simulink model "case9"  (R2024b)
settings: Solver=FixedStepAuto  StartTime=0  StopTime=1  FixedStep=1e-7  RelTol=1e-3
values from neighbouring files (symbols this model uses):
  SG_D_1_D = 0.01056    [IEEE9_case_parameters.m]    (also in case1_parameters.m; case2_parameters.m; case3_parameters.m; case4_parameters.m)
  SG_D_1_EnableSaturation = 0    [IEEE9_case_parameters.m]    (also in case1_parameters.m; case2_parameters.m; case3_parameters.m; case4_parameters.m)
  SG_D_1_f0 = 60    [IEEE9_case_parameters.m]    (also in case1_parameters.m; case2_parameters.m; case3_parameters.m; case4_parameters.m)
  SG_D_1_H = 7.5    [IEEE9_case_parameters.m]    (also in case1_parameters.m; case2_parameters.m; case3_parameters.m; case4_parameters.m)
  SG_D_1_K_A = 20    [IEEE9_case_parameters.m]    (also in case1_parameters.m; case2_parameters.m; case3_parameters.m; case4_parameters.m)
  SG_D_1_K_E = 1.000000e+1    (= 10)    [IEEE9_case_parameters.m]    (also in case1_parameters.m; case2_parameters.m; case3_parameters.m; case4_parameters.m)
  SG_D_1_K_F = 2.363    [IEEE9_case_parameters.m]    (also in case1_parameters.m; case2_parameters.m; case3_parameters.m; case4_parameters.m)
  SG_D_1_K_s = 0.5    [IEEE9_case_parameters.m]    (also in case1_parameters.m = 5; case2_parameters.m = 5; case3_parameters.m = 5; case4_parameters.m = 5)
  SG_D_1_R_a = 0.001088    [IEEE9_case_parameters.m]    (also in case1_parameters.m; case2_parameters.m; case3_parameters.m; case4_parameters.m)
  SG_D_1_S_A = 1    [IEEE9_case_parameters.m]    (also in case1_parameters.m; case2_parameters.m; case3_parameters.m; case4_parameters.m)
  SG_D_1_S_B = 0.103    [IEEE9_case_parameters.m]    (also in case1_parameters.m; case2_parameters.m; case3_parameters.m; case4_parameters.m)
  SG_D_1_S_N = 10.659857    [IEEE9_case_parameters.m]    (also in case1_parameters.m; case2_parameters.m; case3_parameters.m; case4_parameters.m)
  SG_D_1_SpeedPara = 200    [IEEE9_case_parameters.m]    (also in case1_parameters.m; case2_parameters.m; case3_parameters.m; case4_parameters.m)
  SG_D_1_T_0 = 0.720173    [IEEE9_case_parameters.m]    (also in case1_parameters.m = 0.755522; case2_parameters.m = 0.808931; case3_parameters.m = 0.869402; case4_parameters.m = 0.729316)
  SG_D_1_T_1 = 0.3    [IEEE9_case_parameters.m]    (also in case1_parameters.m; case2_parameters.m; case3_parameters.m; case4_parameters.m)
  SG_D_1_T_2 = 0.05    [IEEE9_case_parameters.m]    (also in case1_parameters.m; case2_parameters.m; case3_parameters.m; case4_parameters.m)
  SG_D_1_T_3 = 0.02    [IEEE9_case_parameters.m]    (also in case1_parameters.m; case2_parameters.m; case3_parameters.m; case4_parameters.m)
  SG_D_1_T_4 = 0.005    [IEEE9_case_parameters.m]    (also in case1_parameters.m; case2_parameters.m; case3_parameters.m; case4_parameters.m)
  SG_D_1_T_A = 0.02    [IEEE9_case_parameters.m]    (also in case1_parameters.m; case2_parameters.m; case3_parameters.m; case4_parameters.m)
  SG_D_1_T_dd = 8.000000e+0    (= 8)    [IEEE9_case_parameters.m]    (also in case1_parameters.m; case2_parameters.m; case3_parameters.m; case4_parameters.m)
  SG_D_1_T_ddd = 0.04    [IEEE9_case_parameters.m]    (also in case1_parameters.m; case2_parameters.m; case3_parameters.m; case4_parameters.m)
  SG_D_1_T_E = 0.314    [IEEE9_case_parameters.m]    (also in case1_parameters.m; case2_parameters.m; case3_parameters.m; case4_parameters.m)
  SG_D_1_T_F = 0.35    [IEEE9_case_parameters.m]    (also in case1_parameters.m; case2_parameters.m; case3_parameters.m; case4_parameters.m)
  SG_D_1_T_qd = 0.8    [IEEE9_case_parameters.m]    (also in case1_parameters.m; case2_parameters.m; case3_parameters.m; case4_parameters.m)
  SG_D_1_T_qdd = 0.02    [IEEE9_case_parameters.m]    (also in case1_parameters.m; case2_parameters.m; case3_parameters.m; case4_parameters.m)
  SG_D_1_T_speed = 0.1    [IEEE9_case_parameters.m]    (also in case1_parameters.m = 200; case2_parameters.m = 200; case3_parameters.m = 200; case4_parameters.m = 200)
  SG_D_1_T_w = 0.5    [IEEE9_case_parameters.m]    (also in case1_parameters.m; case2_parameters.m; case3_parameters.m; case4_parameters.m)
  SG_D_1_V_ref = 1.990276    [IEEE9_case_parameters.m]    (also in case1_parameters.m = 2.042296; case2_parameters.m = 2.051388; case3_parameters.m = 2.089584; case4_parameters.m = 2.01845)
  SG_D_1_w_ref = 376.991118    [IEEE9_case_parameters.m]    (also in case1_parameters.m; case2_parameters.m; case3_parameters.m; case4_parameters.m)
  SG_D_1_wb = 6.000000e+1    (= 60)    [IEEE9_case_parameters.m]    (also in case1_parameters.m; case2_parameters.m; case3_parameters.m; case4_parameters.m)
  SG_D_1_x_d = 1.9    [IEEE9_case_parameters.m]    (also in case1_parameters.m; case2_parameters.m; case3_parameters.m; case4_parameters.m)
  SG_D_1_x_dd = 0.302    [IEEE9_case_parameters.m]    (also in case1_parameters.m; case2_parameters.m; case3_parameters.m; case4_parameters.m)
  SG_D_1_x_ddd = 0.204    [IEEE9_case_parameters.m]    (also in case1_parameters.m; case2_parameters.m; case3_parameters.m; case4_parameters.m)
  SG_D_1_x_l = 0.05    [IEEE9_case_parameters.m]    (also in case1_parameters.m; case2_parameters.m; case3_parameters.m; case4_parameters.m)
  SG_D_1_x_q = 1.3    [IEEE9_case_parameters.m]    (also in case1_parameters.m; case2_parameters.m; case3_parameters.m; case4_parameters.m)
  SG_D_1_x_qd = 0.5    [IEEE9_case_parameters.m]    (also in case1_parameters.m; case2_parameters.m; case3_parameters.m; case4_parameters.m)
  SG_D_1_x_qdd = 0.3    [IEEE9_case_parameters.m]    (also in case1_parameters.m; case2_parameters.m; case3_parameters.m; case4_parameters.m)
  SG_D_2_D = 0.02    [IEEE9_case_parameters.m]    (also in case1_parameters.m; case2_parameters.m; case3_parameters.m; case4_parameters.m)
  SG_D_2_EnableSaturation = 0    [IEEE9_case_parameters.m]    (also in case1_parameters.m; case2_parameters.m; case3_parameters.m; case4_parameters.m)
  SG_D_2_f0 = 60    [IEEE9_case_parameters.m]    (also in case1_parameters.m; case2_parameters.m; case3_parameters.m; case4_parameters.m)
  SG_D_2_H = 8.000000e+0    (= 8)    [IEEE9_case_parameters.m]    (also in case1_parameters.m; case2_parameters.m; case3_parameters.m; case4_parameters.m)
  SG_D_2_K_A = 20    [IEEE9_case_parameters.m]    (also in case1_parameters.m; case2_parameters.m; case3_parameters.m; case4_parameters.m)
  SG_D_2_K_E = 1.000000e+1    (= 10)    [IEEE9_case_parameters.m]    (also in case1_parameters.m; case2_parameters.m; case3_parameters.m; case4_parameters.m)
  SG_D_2_K_F = 2.363    [IEEE9_case_parameters.m]    (also in case1_parameters.m; case2_parameters.m; case3_parameters.m; case4_parameters.m)
  SG_D_2_K_s = 0.5    [IEEE9_case_parameters.m]    (also in case1_parameters.m = 4; case2_parameters.m = 4; case3_parameters.m = 4; case4_parameters.m = 4)
  SG_D_2_R_a = 0.001088    [IEEE9_case_parameters.m]    (also in case1_parameters.m; case2_parameters.m; case3_parameters.m; case4_parameters.m)
  SG_D_2_S_A = 1    [IEEE9_case_parameters.m]    (also in case1_parameters.m; case2_parameters.m; case3_parameters.m; case4_parameters.m)
  SG_D_2_S_B = 0.103    [IEEE9_case_parameters.m]    (also in case1_parameters.m; case2_parameters.m; case3_parameters.m; case4_parameters.m)
  SG_D_2_S_N = 10.659857    [IEEE9_case_parameters.m]    (also in case1_parameters.m; case2_parameters.m; case3_parameters.m; case4_parameters.m)
  SG_D_2_SpeedPara = 200    [IEEE9_case_parameters.m]    (also in case1_parameters.m; case2_parameters.m; case3_parameters.m; case4_parameters.m)
  SG_D_2_T_0 = 1.632913    [IEEE9_case_parameters.m]    (also in case1_parameters.m = 1.632925; case2_parameters.m = 1.632915; case3_parameters.m = 1.632914; case4_parameters.m = 1.632927)
  SG_D_2_T_1 = 0.2    [IEEE9_case_parameters.m]    (also in case1_parameters.m; case2_parameters.m; case3_parameters.m; case4_parameters.m)
  SG_D_2_T_2 = 0.05    [IEEE9_case_parameters.m]    (also in case1_parameters.m; case2_parameters.m; case3_parameters.m; case4_parameters.m)
  SG_D_2_T_3 = 0.02    [IEEE9_case_parameters.m]    (also in case1_parameters.m; case2_parameters.m; case3_parameters.m; case4_parameters.m)
  SG_D_2_T_4 = 0.005    [IEEE9_case_parameters.m]    (also in case1_parameters.m; case2_parameters.m; case3_parameters.m; case4_parameters.m)
  SG_D_2_T_A = 0.02    [IEEE9_case_parameters.m]    (also in case1_parameters.m; case2_parameters.m; case3_parameters.m; case4_parameters.m)
  SG_D_2_T_dd = 7.9    [IEEE9_case_parameters.m]    (also in case1_parameters.m; case2_parameters.m; case3_parameters.m; case4_parameters.m)
  SG_D_2_T_ddd = 0.04    [IEEE9_case_parameters.m]    (also in case1_parameters.m; case2_parameters.m; case3_parameters.m; case4_parameters.m)
  SG_D_2_T_E = 0.314    [IEEE9_case_parameters.m]    (also in case1_parameters.m; case2_parameters.m; case3_parameters.m; case4_parameters.m)
  SG_D_2_T_F = 0.35    [IEEE9_case_parameters.m]    (also in case1_parameters.m; case2_parameters.m; case3_parameters.m; case4_parameters.m)
  SG_D_2_T_qd = 0.8    [IEEE9_case_parameters.m]    (also in case1_parameters.m; case2_parameters.m; case3_parameters.m; case4_parameters.m)
  SG_D_2_T_qdd = 0.015    [IEEE9_case_parameters.m]    (also in case1_parameters.m; case2_parameters.m; case3_parameters.m; case4_parameters.m)
  SG_D_2_T_speed = 0.1    [IEEE9_case_parameters.m]    (also in case1_parameters.m = 150; case2_parameters.m = 150; case3_parameters.m = 150; case4_parameters.m = 150)
  SG_D_2_T_w = 0.35    [IEEE9_case_parameters.m]    (also in case1_parameters.m; case2_parameters.m; case3_parameters.m; case4_parameters.m)
  SG_D_2_V_ref = 2.58547    [IEEE9_case_parameters.m]    (also in case1_parameters.m = 2.597896; case2_parameters.m = 2.587136; case3_parameters.m = 2.586042; case4_parameters.m = 2.599679)
  SG_D_2_w_ref = 376.991118    [IEEE9_case_parameters.m]    (also in case1_parameters.m; case2_parameters.m; case3_parameters.m; case4_parameters.m)
  SG_D_2_wb = 6.000000e+1    (= 60)    [IEEE9_case_parameters.m]    (also in case1_parameters.m; case2_parameters.m; case3_parameters.m; case4_parameters.m)
  SG_D_2_x_d = 1.8    [IEEE9_case_parameters.m]    (also in case1_parameters.m; case2_parameters.m; case3_parameters.m; case4_parameters.m)
  SG_D_2_x_dd = 0.302    [IEEE9_case_parameters.m]    (also in case1_parameters.m; case2_parameters.m; case3_parameters.m; case4_parameters.m)
  SG_D_2_x_ddd = 0.204    [IEEE9_case_parameters.m]    (also in case1_parameters.m; case2_parameters.m; case3_parameters.m; case4_parameters.m)
  SG_D_2_x_l = 0.05    [IEEE9_case_parameters.m]    (also in case1_parameters.m; case2_parameters.m; case3_parameters.m; case4_parameters.m)
  SG_D_2_x_q = 1.25    [IEEE9_case_parameters.m]    (also in case1_parameters.m; case2_parameters.m; case3_parameters.m; case4_parameters.m)
  SG_D_2_x_qd = 0.5    [IEEE9_case_parameters.m]    (also in case1_parameters.m; case2_parameters.m; case3_parameters.m; case4_parameters.m)
  SG_D_2_x_qdd = 0.3    [IEEE9_case_parameters.m]    (also in case1_parameters.m; case2_parameters.m; case3_parameters.m; case4_parameters.m)
  SG_D_3_D = 0.02    [IEEE9_case_parameters.m]    (also in case1_parameters.m; case2_parameters.m; case3_parameters.m; case4_parameters.m)
  SG_D_3_EnableSaturation = 0    [IEEE9_case_parameters.m]    (also in case1_parameters.m; case2_parameters.m; case3_parameters.m; case4_parameters.m)
  SG_D_3_f0 = 60    [IEEE9_case_parameters.m]    (also in case1_parameters.m; case2_parameters.m; case3_parameters.m; case4_parameters.m)
  SG_D_3_H = 7.7    [IEEE9_case_parameters.m]    (also in case1_parameters.m; case2_parameters.m; case3_parameters.m; case4_parameters.m)
  SG_D_3_K_A = 20    [IEEE9_case_parameters.m]    (also in case1_parameters.m; case2_parameters.m; case3_parameters.m; case4_parameters.m)
  SG_D_3_K_E = 1.000000e+1    (= 10)    [IEEE9_case_parameters.m]    (also in case1_parameters.m; case2_parameters.m; case3_parameters.m; case4_parameters.m)
  SG_D_3_K_F = 2.363    [IEEE9_case_parameters.m]    (also in case1_parameters.m; case2_parameters.m; case3_parameters.m; case4_parameters.m)
  SG_D_3_K_s = 0.2    [IEEE9_case_parameters.m]    (also in case1_parameters.m = 2; case2_parameters.m = 2; case3_parameters.m = 2; case4_parameters.m = 2)
  SG_D_3_R_a = 0.001088    [IEEE9_case_parameters.m]    (also in case1_parameters.m; case2_parameters.m; case3_parameters.m; case4_parameters.m)
  SG_D_3_S_A = 1    [IEEE9_case_parameters.m]    (also in case1_parameters.m; case2_parameters.m; case3_parameters.m; case4_parameters.m)
  SG_D_3_S_B = 0.103    [IEEE9_case_parameters.m]    (also in case1_parameters.m; case2_parameters.m; case3_parameters.m; case4_parameters.m)
  SG_D_3_S_N = 10.659857    [IEEE9_case_parameters.m]    (also in case1_parameters.m; case2_parameters.m; case3_parameters.m; case4_parameters.m)
  SG_D_3_SpeedPara = 200    [IEEE9_case_parameters.m]    (also in case1_parameters.m; case2_parameters.m; case3_parameters.m; case4_parameters.m)
  SG_D_3_T_0 = 0.850788    [IEEE9_case_parameters.m]    (also in case1_parameters.m = 0.850786; case2_parameters.m = 0.850787; case3_parameters.m; case4_parameters.m = 0.850786)
  SG_D_3_T_1 = 0.2    [IEEE9_case_parameters.m]    (also in case1_parameters.m; case2_parameters.m; case3_parameters.m; case4_parameters.m)
  SG_D_3_T_2 = 0.05    [IEEE9_case_parameters.m]    (also in case1_parameters.m; case2_parameters.m; case3_parameters.m; case4_parameters.m)
  SG_D_3_T_3 = 0.02    [IEEE9_case_parameters.m]    (also in case1_parameters.m; case2_parameters.m; case3_parameters.m; case4_parameters.m)
  SG_D_3_T_4 = 0.005    [IEEE9_case_parameters.m]    (also in case1_parameters.m; case2_parameters.m; case3_parameters.m; case4_parameters.m)
  SG_D_3_T_A = 0.02    [IEEE9_case_parameters.m]    (also in case1_parameters.m; case2_parameters.m; case3_parameters.m; case4_parameters.m)
  SG_D_3_T_dd = 8.1    [IEEE9_case_parameters.m]    (also in case1_parameters.m; case2_parameters.m; case3_parameters.m; case4_parameters.m)
  SG_D_3_T_ddd = 0.04    [IEEE9_case_parameters.m]    (also in case1_parameters.m; case2_parameters.m; case3_parameters.m; case4_parameters.m)
  SG_D_3_T_E = 0.314    [IEEE9_case_parameters.m]    (also in case1_parameters.m; case2_parameters.m; case3_parameters.m; case4_parameters.m)
  SG_D_3_T_F = 0.35    [IEEE9_case_parameters.m]    (also in case1_parameters.m; case2_parameters.m; case3_parameters.m; case4_parameters.m)
  SG_D_3_T_qd = 0.8    [IEEE9_case_parameters.m]    (also in case1_parameters.m; case2_parameters.m; case3_parameters.m; case4_parameters.m)
  SG_D_3_T_qdd = 0.015    [IEEE9_case_parameters.m]    (also in case1_parameters.m; case2_parameters.m; case3_parameters.m; case4_parameters.m)
  SG_D_3_T_speed = 0.1    [IEEE9_case_parameters.m]    (also in case1_parameters.m = 180; case2_parameters.m = 180; case3_parameters.m = 180; case4_parameters.m = 180)
  SG_D_3_T_w = 0.4    [IEEE9_case_parameters.m]    (also in case1_parameters.m; case2_parameters.m; case3_parameters.m; case4_parameters.m)
  SG_D_3_V_ref = 1.892727    [IEEE9_case_parameters.m]    (also in case1_parameters.m = 1.906439; case2_parameters.m = 1.895535; case3_parameters.m = 1.892105; case4_parameters.m = 1.906598)
  SG_D_3_w_ref = 376.991118    [IEEE9_case_parameters.m]    (also in case1_parameters.m; case2_parameters.m; case3_parameters.m; case4_parameters.m)
  SG_D_3_wb = 6.000000e+1    (= 60)    [IEEE9_case_parameters.m]    (also in case1_parameters.m; case2_parameters.m; case3_parameters.m; case4_parameters.m)
  SG_D_3_x_d = 1.85    [IEEE9_case_parameters.m]    (also in case1_parameters.m; case2_parameters.m; case3_parameters.m; case4_parameters.m)
  SG_D_3_x_dd = 0.302    [IEEE9_case_parameters.m]    (also in case1_parameters.m; case2_parameters.m; case3_parameters.m; case4_parameters.m)
  SG_D_3_x_ddd = 0.204    [IEEE9_case_parameters.m]    (also in case1_parameters.m; case2_parameters.m; case3_parameters.m; case4_parameters.m)
  SG_D_3_x_l = 0.05    [IEEE9_case_parameters.m]    (also in case1_parameters.m; case2_parameters.m; case3_parameters.m; case4_parameters.m)
  SG_D_3_x_q = 1.2    [IEEE9_case_parameters.m]    (also in case1_parameters.m; case2_parameters.m; case3_parameters.m; case4_parameters.m)
  SG_D_3_x_qd = 0.5    [IEEE9_case_parameters.m]    (also in case1_parameters.m; case2_parameters.m; case3_parameters.m; case4_parameters.m)
  SG_D_3_x_qdd = 0.3    [IEEE9_case_parameters.m]    (also in case1_parameters.m; case2_parameters.m; case3_parameters.m; case4_parameters.m)
(part 8 of 12)

== system case9/Apparatus/SG_D_2/d_psi_1d_SG_D_2_block ==
  note: d_psi_1d_SG_D_2 in case9
      | $-\frac{\psi _{\mathrm{1d},\mathrm{SG},D,2}-\psi _{\mathrm{fd},\mathrm{SG},D,2}+\frac{\left(x_{\mathrm{dd}}-x_{l}\right)\,\left(\frac{\psi _{\mathrm{1d},\mathrm{SG},D,2}\,\left(x_{\mathrm{dd}}-x_{\mathrm{ddd}}\right)}{x_{\mathrm{dd}}-x_{l}}-\psi _{d,\mathrm{SG},D,2}+\frac{\psi _{\mathrm{fd},\mathrm{SG},D,2}\,\left(x_{\mathrm{ddd}}-x_{l}\right)}{x_{\mathrm{dd}}-x_{l}}\right)}{x_{\mathrm{ddd}}}}{T_{\mathrm{ddd}}}$
      | Automatically generated on 2025-10-31 19:34:57 .
  State_psi_1d_SG_D_2_9b1ac : Inport
  State_psi_fd_SG_D_2_31ac8 : Inport  Port=2
  State_psi_1d_SG_D_2_4f306 : Inport  Port=3
  State_psi_d_SG_D_2_6c073 : Inport  Port=4
  State_psi_fd_SG_D_2_e2670 : Inport  Port=5
  Add_18fc3 : Sum
  Add_47703 : Sum
  Add_7959e : Sum
  Constant_-1_6db51 : Constant  Value=-1
  Constant_-1_c8e40 : Constant  Value=-1
  Constant_T_ddd_9bdcc : Constant  Value=T_ddd
  Constant_x_dd_6105a : Constant  Value=x_dd
  Constant_x_dd_8007f : Constant  Value=x_dd
  Constant_x_dd_b55d8 : Constant  Value=x_dd
  Constant_x_dd_ce09f : Constant  Value=x_dd
  Constant_x_ddd_0d417 : Constant  Value=x_ddd
  Constant_x_ddd_3c9c5 : Constant  Value=x_ddd
  Constant_x_ddd_7b55f : Constant  Value=x_ddd
  Constant_x_l_30dfb : Constant  Value=x_l
  Constant_x_l_5fcac : Constant  Value=x_l
  Constant_x_l_78aaf : Constant  Value=x_l
  Constant_x_l_b2922 : Constant  Value=x_l
  Divide_0f227 : Product  Inputs=*/
  Divide_c3476 : Product  Inputs=*/
  Divide_d66d9 : Product  Inputs=*/
  Divide_de240 : Product  Inputs=*/
  Product_030dc : Product
  Product_0f4d7 : Product
  Product_2a33a : Product
  Product_5af6c : Product
  Product_d701c : Product
  Subtract_1056e : Sum  Inputs=+-
  Subtract_1b7e0 : Sum  Inputs=+-
  Subtract_67225 : Sum  Inputs=+-
  Subtract_7c716 : Sum  Inputs=+-
  Subtract_a97c8 : Sum  Inputs=+-
  Subtract_cfbe6 : Sum  Inputs=+-
  Blockout_d_psi_1d_SG_D_2_4d013 : Outport
  wires:
  Subtract_67225/1 -> Product_5af6c/2
  Constant_x_l_b2922/1 -> Subtract_a97c8/2
  Divide_0f227/1 -> Add_47703/2
  Subtract_1b7e0/1 -> Product_d701c/2
  Constant_-1_c8e40/1 -> Product_0f4d7/1
  Constant_x_dd_8007f/1 -> Subtract_1056e/1
  Divide_c3476/1 -> Blockout_d_psi_1d_SG_D_2_4d013/1
  State_psi_fd_SG_D_2_31ac8/1 -> Add_7959e/2
  State_psi_1d_SG_D_2_4f306/1 -> Product_0f4d7/2
  Divide_de240/1 -> Subtract_1b7e0/2
  Constant_x_ddd_3c9c5/1 -> Subtract_1056e/2
  State_psi_1d_SG_D_2_9b1ac/1 -> Product_030dc/2
  Product_0f4d7/1 -> Product_2a33a/1
  Subtract_1056e/1 -> Product_2a33a/2
  Constant_x_dd_b55d8/1 -> Subtract_a97c8/1
  Constant_x_ddd_0d417/1 -> Subtract_67225/1
  Constant_x_l_5fcac/1 -> Subtract_67225/2
  Product_2a33a/1 -> Divide_d66d9/1
  Subtract_a97c8/1 -> Divide_d66d9/2
  State_psi_fd_SG_D_2_e2670/1 -> Product_5af6c/1
  Constant_x_dd_ce09f/1 -> Subtract_cfbe6/1
  Constant_x_l_78aaf/1 -> Subtract_7c716/2
  Constant_x_l_30dfb/1 -> Subtract_cfbe6/2
  Constant_x_ddd_7b55f/1 -> Divide_0f227/2
  Divide_d66d9/1 -> Add_18fc3/1
  State_psi_d_SG_D_2_6c073/1 -> Add_18fc3/2
  Product_5af6c/1 -> Divide_de240/1
  Subtract_cfbe6/1 -> Divide_de240/2
  Constant_x_dd_6105a/1 -> Subtract_7c716/1
  Add_18fc3/1 -> Subtract_1b7e0/1
  Constant_-1_6db51/1 -> Product_030dc/1
  Subtract_7c716/1 -> Product_d701c/1
  Product_030dc/1 -> Add_7959e/1
  Product_d701c/1 -> Divide_0f227/1
  Add_7959e/1 -> Add_47703/1
  Add_47703/1 -> Divide_c3476/1
  Constant_T_ddd_9bdcc/1 -> Divide_c3476/2

== system case9/Apparatus/SG_D_2/d_psi_d_SG_D_2_block ==
  note: d_psi_d_SG_D_2 in case9
      | $2\,\pi \,f_{0}\,\left(v_{d,\mathrm{SG},D,2}\,\sin\left(\theta _{\mathrm{SG},D,2}\right)-v_{q,\mathrm{SG},D,2}\,\cos\left(\theta _{\mathrm{SG},D,2}\right)+\frac{R_{a}\,\left(\frac{\psi _{\mathrm{1d},\mathrm{SG},D,2}\,\left(x_{\mathrm{dd}}-x_{\mathrm{ddd}}\right)}{x_{\mathrm{dd}}-x_{l}}-\psi _{d,\mathrm{SG},D,2}+\frac{\psi _{\mathrm{fd},\mathrm{SG},D,2}\,\left(x_{\mathrm{ddd}}-x_{l}\right)}{x_{\mathrm{dd}}-x_{l}}\right)}{x_{\mathrm{ddd}}}+\frac{\psi _{q,\mathrm{SG},D,2}\,w_{\mathrm{SG},D,2}}{2\,f_{0}\,\pi }\right)$
      | Automatically generated on 2025-10-31 19:34:54 .
  State_psi_1d_SG_D_2_d40cf : Inport
  State_psi_d_SG_D_2_25359 : Inport  Port=2
  State_psi_fd_SG_D_2_9b2f4 : Inport  Port=3
  Input_v_d_SG_D_2_d9ecd : Inport  Port=4
  State_theta_SG_D_2_7b7d1 : Inport  Port=5
  Input_v_q_SG_D_2_cb8d6 : Inport  Port=6
  State_theta_SG_D_2_ed5aa : Inport  Port=7
  State_psi_q_SG_D_2_78b00 : Inport  Port=8
  State_w_SG_D_2_fe89e : Inport  Port=9
  Add_1e130 : Sum
  Add_95736 : Sum
  Constant_-1_d1a72 : Constant  Value=-1
  Constant_-2.0_0a84b : Constant  Value=-2.0
  Constant_2.0_16524 : Constant  Value=2.0
  Constant_R_a_5fe79 : Constant  Value=R_a
  Constant_f0_c8b30 : Constant  Value=f0
  Constant_f0_d903e : Constant  Value=f0
  Constant_pi_38b7b : Constant  Value=pi
  Constant_pi_4bdac : Constant  Value=pi
  Constant_x_dd_2b82b : Constant  Value=x_dd
  Constant_x_dd_8fa44 : Constant  Value=x_dd
  Constant_x_dd_f8b5d : Constant  Value=x_dd
  Constant_x_ddd_0f6ba : Constant  Value=x_ddd
  Constant_x_ddd_d2d74 : Constant  Value=x_ddd
  Constant_x_ddd_e65f6 : Constant  Value=x_ddd
  Constant_x_l_65b5e : Constant  Value=x_l
  Constant_x_l_931b8 : Constant  Value=x_l
  Constant_x_l_af2d2 : Constant  Value=x_l
  Divide_2b745 : Product  Inputs=*/
  Divide_6bfed : Product  Inputs=*/
  Divide_c59a3 : Product  Inputs=*/
  Divide_ca9bb : Product  Inputs=*/
  MathFunc_cos_be2da : Trigonometry  Operator=cos
  MathFunc_sin_18cab : Trigonometry
  Product_0fb18 : Product
  Product_2a09d : Product
  Product_2f75e : Product
  Product_37f48 : Product
  Product_64ad8 : Product
  Product_6754d : Product
  Product_7a1cc : Product
  Product_a149a : Product
  Product_d38ff : Product
  Product_daf8b : Product
  Product_dd7d7 : Product
  Product_e1648 : Product
  Subtract_1b078 : Sum  Inputs=+-
  Subtract_24d92 : Sum  Inputs=+-
  Subtract_b40c2 : Sum  Inputs=+-
  Subtract_c682e : Sum  Inputs=+-
  Subtract_ccaed : Sum  Inputs=+-
  Subtract_e850a : Sum  Inputs=+-
  Subtract_f83ea : Sum  Inputs=+-
  Blockout_d_psi_d_SG_D_2_17d26 : Outport
  wires:
  MathFunc_sin_18cab/1 -> Product_e1648/2
  Constant_x_dd_f8b5d/1 -> Subtract_e850a/1
  Constant_-1_d1a72/1 -> Product_2f75e/1
  Constant_x_l_931b8/1 -> Subtract_e850a/2
  State_psi_1d_SG_D_2_d40cf/1 -> Product_2f75e/2
  Constant_f0_c8b30/1 -> Product_d38ff/2
  Constant_2.0_16524/1 -> Product_64ad8/1
  Constant_x_l_af2d2/1 -> Subtract_ccaed/2
  Constant_x_dd_2b82b/1 -> Subtract_24d92/1
  Product_2a09d/1 -> Blockout_d_psi_d_SG_D_2_17d26/1
  Constant_pi_38b7b/1 -> Product_64ad8/2
  Constant_x_ddd_e65f6/1 -> Subtract_24d92/2
  Subtract_1b078/1 -> Product_2a09d/2
  Product_2f75e/1 -> Product_6754d/1
  Product_64ad8/1 -> Product_7a1cc/1
  Subtract_24d92/1 -> Product_6754d/2
  Divide_ca9bb/1 -> Subtract_1b078/2
  Constant_x_ddd_d2d74/1 -> Subtract_b40c2/1
  Constant_x_l_65b5e/1 -> Subtract_b40c2/2
  Product_6754d/1 -> Divide_2b745/1
  Subtract_f83ea/1 -> Add_1e130/1
  Subtract_e850a/1 -> Divide_2b745/2
  State_psi_fd_SG_D_2_9b2f4/1 -> Product_daf8b/1
  Subtract_b40c2/1 -> Product_daf8b/2
  Constant_x_dd_8fa44/1 -> Subtract_ccaed/1
  Divide_2b745/1 -> Add_95736/1
  State_psi_d_SG_D_2_25359/1 -> Add_95736/2
  Product_daf8b/1 -> Divide_c59a3/1
  Subtract_ccaed/1 -> Divide_c59a3/2
  Add_95736/1 -> Subtract_c682e/1
  Divide_c59a3/1 -> Subtract_c682e/2
  Constant_R_a_5fe79/1 -> Product_0fb18/1
  Subtract_c682e/1 -> Product_0fb18/2
  Divide_6bfed/1 -> Subtract_f83ea/1
  State_theta_SG_D_2_7b7d1/1 -> MathFunc_sin_18cab/1
  Product_0fb18/1 -> Divide_6bfed/1
  Constant_-2.0_0a84b/1 -> Product_dd7d7/1
  Input_v_d_SG_D_2_d9ecd/1 -> Product_e1648/1
  Constant_x_ddd_0f6ba/1 -> Divide_6bfed/2
  State_theta_SG_D_2_ed5aa/1 -> MathFunc_cos_be2da/1
  Product_d38ff/1 -> Product_2a09d/1
  Product_e1648/1 -> Subtract_f83ea/2
  Product_dd7d7/1 -> Product_d38ff/1
  Input_v_q_SG_D_2_cb8d6/1 -> Product_37f48/1
  MathFunc_cos_be2da/1 -> Product_37f48/2
  State_psi_q_SG_D_2_78b00/1 -> Product_a149a/1
  State_w_SG_D_2_fe89e/1 -> Product_a149a/2
  Constant_f0_d903e/1 -> Product_7a1cc/2
  Constant_pi_4bdac/1 -> Product_dd7d7/2
  Product_37f48/1 -> Add_1e130/2
  Product_a149a/1 -> Divide_ca9bb/1
  Product_7a1cc/1 -> Divide_ca9bb/2
  Add_1e130/1 -> Subtract_1b078/1

== system case9/Apparatus/SG_D_2/d_psi_fd_SG_D_2_block ==
  note: d_psi_fd_SG_D_2 in case9
      | $-\frac{\psi _{\mathrm{fd},\mathrm{SG},D,2}-E_{\mathrm{fd},\mathrm{SG},D,2}+\left(x_{d}-x_{\mathrm{dd}}\right)\,\left(\frac{\frac{\psi _{\mathrm{1d},\mathrm{SG},D,2}\,\left(x_{\mathrm{dd}}-x_{\mathrm{ddd}}\right)}{x_{\mathrm{dd}}-x_{l}}-\psi _{d,\mathrm{SG},D,2}+\frac{\psi _{\mathrm{fd},\mathrm{SG},D,2}\,\left(x_{\mathrm{ddd}}-x_{l}\right)}{x_{\mathrm{dd}}-x_{l}}}{x_{\mathrm{ddd}}}-\frac{\left(x_{\mathrm{dd}}-x_{\mathrm{ddd}}\right)\,\left(\psi _{\mathrm{1d},\mathrm{SG},D,2}-\psi _{\mathrm{fd},\mathrm{SG},D,2}+\frac{\left(x_{\mathrm{dd}}-x_{l}\right)\,\left(\frac{\psi _{\mathrm{1d},\mathrm{SG},D,2}\,\left(x_{\mathrm{dd}}-x_{\mathrm{ddd}}\right)}{x_{\mathrm{dd}}-x_{l}}-\psi _{d,\mathrm{SG},D,2}+\frac{\psi _{\mathrm{fd},\mathrm{SG},D,2}\,\left(x_{\mathrm{ddd}}-x_{l}\right)}{x_{\mathrm{dd}}-x_{l}}\right)}{x_{\mathrm{ddd}}}\right)}{{\left(x_{\mathrm{dd}}-x_{l}\right)}^2}\right)}{T_{\mathrm{dd}}}$
      | Automatically generated on 2025-10-31 19:34:56 .
  State_E_fd_SG_D_2_5eccf : Inport
  State_psi_fd_SG_D_2_a7474 : Inport  Port=2
  State_psi_1d_SG_D_2_eaed7 : Inport  Port=3
  State_psi_fd_SG_D_2_5a6db : Inport  Port=4
  State_psi_1d_SG_D_2_c8d95 : Inport  Port=5
  State_psi_d_SG_D_2_a4024 : Inport  Port=6
  State_psi_fd_SG_D_2_151d3 : Inport  Port=7
  State_psi_1d_SG_D_2_fe5ae : Inport  Port=8
  State_psi_d_SG_D_2_cc219 : Inport  Port=9
  State_psi_fd_SG_D_2_1d8e3 : Inport  Port=10
  Add_676fd : Sum
  Add_809fa : Sum
  Constant_-1_955d1 : Constant  Value=-1
  Constant_-1_b7711 : Constant  Value=-1
  Constant_-1_bdc37 : Constant  Value=-1
  Constant_2.0_6795e : Constant  Value=2.0
  Constant_T_dd_c2ebe : Constant  Value=T_dd
  Constant_x_d_21a87 : Constant  Value=x_d
  Constant_x_dd_0c06f : Constant  Value=x_dd
  Constant_x_dd_1efb2 : Constant  Value=x_dd
  Constant_x_dd_3f41e : Constant  Value=x_dd
  Constant_x_dd_5792a : Constant  Value=x_dd
  Constant_x_dd_5f4b2 : Constant  Value=x_dd
  Constant_x_dd_657cb : Constant  Value=x_dd
  Constant_x_dd_687e3 : Constant  Value=x_dd
  Constant_x_dd_7842e : Constant  Value=x_dd
  Constant_x_dd_bf877 : Constant  Value=x_dd
  Constant_x_dd_d26d9 : Constant  Value=x_dd
  Constant_x_ddd_16458 : Constant  Value=x_ddd
  Constant_x_ddd_36004 : Constant  Value=x_ddd
  Constant_x_ddd_567b5 : Constant  Value=x_ddd
  Constant_x_ddd_7a9a3 : Constant  Value=x_ddd
  Constant_x_ddd_82ded : Constant  Value=x_ddd
  Constant_x_ddd_98200 : Constant  Value=x_ddd
  Constant_x_ddd_a2be3 : Constant  Value=x_ddd
  Constant_x_l_0f469 : Constant  Value=x_l
  Constant_x_l_13f2f : Constant  Value=x_l
  Constant_x_l_1c729 : Constant  Value=x_l
  Constant_x_l_2b70b : Constant  Value=x_l
  Constant_x_l_942a5 : Constant  Value=x_l
  Constant_x_l_ad6ed : Constant  Value=x_l
  Constant_x_l_b7b1d : Constant  Value=x_l
  Constant_x_l_c350b : Constant  Value=x_l
  Divide_290ff : Product  Inputs=*/
  Divide_583e5 : Product  Inputs=*/
  Divide_5f973 : Product  Inputs=*/
  Divide_6e344 : Product  Inputs=*/
  Divide_99481 : Product  Inputs=*/
  Divide_ce59d : Product  Inputs=*/
  Divide_d665e : Product  Inputs=*/
  Divide_fe53e : Product  Inputs=*/
  Power_5a083 : Math  Operator=pow
  Product_32dd5 : Product
  Product_34916 : Product
  Product_6c795 : Product
  Product_7516a : Product
  Product_7d71a : Product
  Product_a290e : Product
  Product_bd735 : Product
  Product_c09a7 : Product
  Product_e2bbc : Product
  Product_fd7d8 : Product
  Subtract_0377f : Sum  Inputs=+-
  Subtract_05f48 : Sum  Inputs=+-
  Subtract_1895f : Sum  Inputs=+-
  Subtract_1ab2a : Sum  Inputs=+-
  Subtract_1dd1f : Sum  Inputs=+-
  Subtract_3a82e : Sum  Inputs=+-
  Subtract_6ca6b : Sum  Inputs=+-
  Subtract_6db93 : Sum  Inputs=+-
  Subtract_74dc5 : Sum  Inputs=+-
  Subtract_8c2c0 : Sum  Inputs=+-
  Subtract_a2730 : Sum  Inputs=+-
  Subtract_a6d5d : Sum  Inputs=+-
  Subtract_aab37 : Sum  Inputs=+-
  Subtract_ad48d : Sum  Inputs=+-
  Subtract_bd0a5 : Sum  Inputs=+-
  Subtract_bf7ad : Sum  Inputs=+-
  Subtract_d44dc : Sum  Inputs=+-
  Subtract_df81d : Sum  Inputs=+-
  Subtract_fab20 : Sum  Inputs=+-
  Blockout_d_psi_fd_SG_D_2_bffd5 : Outport
  wires:
  Constant_x_dd_bf877/1 -> Subtract_1ab2a/1
  Constant_-1_b7711/1 -> Product_34916/1
  Constant_x_l_1c729/1 -> Subtract_8c2c0/2
  Divide_ce59d/1 -> Add_809fa/1
  Subtract_0377f/1 -> Product_7516a/2
  Constant_x_l_b7b1d/1 -> Subtract_1ab2a/2
  Product_7516a/1 -> Divide_6e344/1
  State_psi_1d_SG_D_2_c8d95/1 -> Product_34916/2
  Constant_x_dd_657cb/1 -> Subtract_6ca6b/1
  Product_c09a7/1 -> Divide_ce59d/1
  Constant_x_dd_0c06f/1 -> Subtract_ad48d/1
  Constant_x_ddd_7a9a3/1 -> Subtract_6ca6b/2
  Constant_x_dd_3f41e/1 -> Subtract_6db93/1
  Product_34916/1 -> Product_7d71a/1
  Subtract_6ca6b/1 -> Product_7d71a/2
  State_psi_d_SG_D_2_cc219/1 -> Add_809fa/2
  Constant_x_ddd_567b5/1 -> Subtract_0377f/1
  Constant_x_l_ad6ed/1 -> Subtract_0377f/2
  Product_7d71a/1 -> Divide_d665e/1
  Subtract_1ab2a/1 -> Divide_d665e/2
  State_psi_fd_SG_D_2_151d3/1 -> Product_7516a/1
  Subtract_bd0a5/1 -> Product_e2bbc/2
  Constant_x_dd_5792a/1 -> Subtract_05f48/1
  Constant_x_l_942a5/1 -> Subtract_05f48/2
  Product_a290e/1 -> Product_e2bbc/1
  Divide_d665e/1 -> Add_676fd/1
  State_psi_d_SG_D_2_a4024/1 -> Add_676fd/2
  Subtract_05f48/1 -> Divide_6e344/2
  Constant_x_dd_5f4b2/1 -> Subtract_8c2c0/1
  Constant_x_ddd_36004/1 -> Subtract_1dd1f/1
  Add_676fd/1 -> Subtract_74dc5/1
  Divide_6e344/1 -> Subtract_74dc5/2
  Constant_-1_bdc37/1 -> Product_32dd5/1
  Product_fd7d8/1 -> Divide_99481/1
  State_psi_1d_SG_D_2_fe5ae/1 -> Product_32dd5/2
  Subtract_ad48d/1 -> Product_a290e/2
  Constant_x_dd_1efb2/1 -> Subtract_aab37/1
  Divide_99481/1 -> Subtract_a6d5d/2
  Constant_-1_955d1/1 -> Product_a290e/1
  Constant_x_ddd_98200/1 -> Subtract_aab37/2
  Constant_x_ddd_16458/1 -> Divide_fe53e/2
  Subtract_8c2c0/1 -> Product_6c795/1
  Subtract_74dc5/1 -> Product_6c795/2
  State_psi_fd_SG_D_2_5a6db/1 -> Subtract_1895f/2
  Product_32dd5/1 -> Product_c09a7/1
  Subtract_aab37/1 -> Product_c09a7/2
  Constant_2.0_6795e/1 -> Power_5a083/2
  State_psi_1d_SG_D_2_eaed7/1 -> Subtract_1895f/1
  Constant_x_dd_d26d9/1 -> Subtract_d44dc/1
  Subtract_1dd1f/1 -> Product_fd7d8/2
  Constant_x_l_13f2f/1 -> Subtract_d44dc/2
  Constant_x_l_c350b/1 -> Subtract_1dd1f/2
  Constant_x_ddd_82ded/1 -> Subtract_ad48d/2
  Subtract_6db93/1 -> Divide_99481/2
  Product_6c795/1 -> Divide_fe53e/1
  Subtract_d44dc/1 -> Divide_ce59d/2
  State_psi_fd_SG_D_2_1d8e3/1 -> Product_fd7d8/1
  Constant_x_l_2b70b/1 -> Subtract_6db93/2
  Constant_x_dd_687e3/1 -> Subtract_bf7ad/1
  Subtract_1895f/1 -> Subtract_bd0a5/1
  Divide_fe53e/1 -> Subtract_bd0a5/2
  Constant_x_l_0f469/1 -> Subtract_bf7ad/2
  Subtract_bf7ad/1 -> Power_5a083/1
  Add_809fa/1 -> Subtract_a6d5d/1
  Product_e2bbc/1 -> Divide_290ff/1
  Power_5a083/1 -> Divide_290ff/2
  Subtract_a6d5d/1 -> Divide_5f973/1
  Constant_x_ddd_a2be3/1 -> Divide_5f973/2
  Constant_x_d_21a87/1 -> Subtract_fab20/1
  Constant_x_dd_7842e/1 -> Subtract_fab20/2
  Divide_290ff/1 -> Subtract_3a82e/1
  Divide_5f973/1 -> Subtract_3a82e/2
  State_E_fd_SG_D_2_5eccf/1 -> Subtract_a2730/1
  State_psi_fd_SG_D_2_a7474/1 -> Subtract_a2730/2
  Subtract_fab20/1 -> Product_bd735/1
  Subtract_3a82e/1 -> Product_bd735/2
  Subtract_a2730/1 -> Subtract_df81d/1
  Product_bd735/1 -> Subtract_df81d/2
  Subtract_df81d/1 -> Divide_583e5/1
  Constant_T_dd_c2ebe/1 -> Divide_583e5/2
  Divide_583e5/1 -> Blockout_d_psi_fd_SG_D_2_bffd5/1

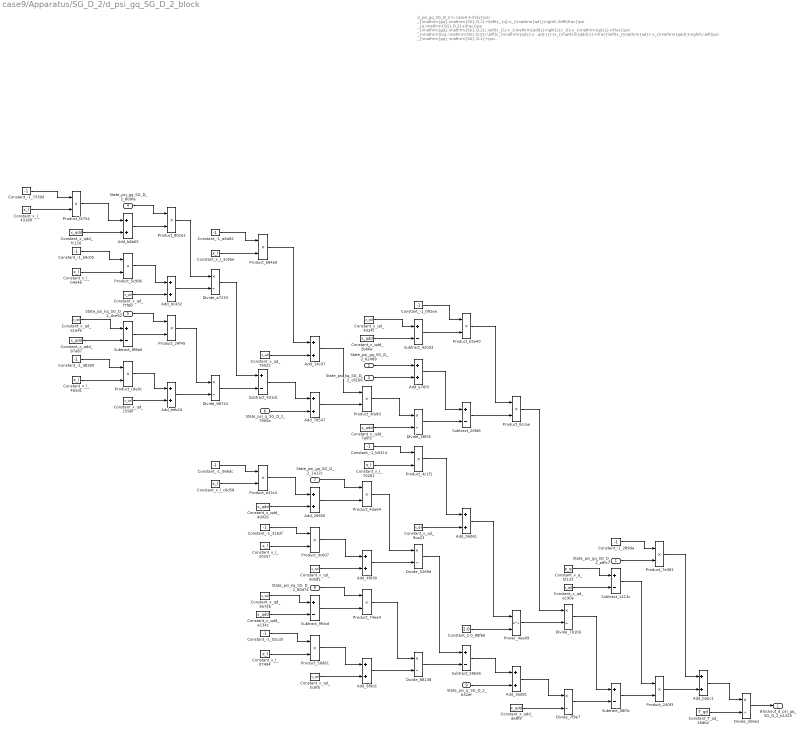
== system case9/Apparatus/SG_D_2/d_psi_gq_SG_D_2_block ==
  note: d_psi_gq_SG_D_2 in case9
      | $-\frac{\psi _{\mathrm{gq},\mathrm{SG},D,2}+\left(x_{q}-x_{\mathrm{qd}}\right)\,\left(\frac{\psi _{q,\mathrm{SG},D,2}+\frac{\psi _{\mathrm{gq},\mathrm{SG},D,2}\,\left(x_{l}-x_{\mathrm{qdd}}\right)}{x_{l}-x_{\mathrm{qd}}}+\frac{\psi _{\mathrm{kq},\mathrm{SG},D,2}\,\left(x_{\mathrm{qd}}-x_{\mathrm{qdd}}\right)}{x_{l}-x_{\mathrm{qd}}}}{x_{\mathrm{qdd}}}+\frac{\left(x_{\mathrm{qd}}-x_{\mathrm{qdd}}\right)\,\left(\psi _{\mathrm{gq},\mathrm{SG},D,2}+\psi _{\mathrm{kq},\mathrm{SG},D,2}+\frac{\left(x_{l}-x_{\mathrm{qd}}\right)\,\left(\psi _{q,\mathrm{SG},D,2}+\frac{\psi _{\mathrm{gq},\mathrm{SG},D,2}\,\left(x_{l}-x_{\mathrm{qdd}}\right)}{x_{l}-x_{\mathrm{qd}}}+\frac{\psi _{\mathrm{kq},\mathrm{SG},D,2}\,\left(x_{\mathrm{qd}}-x_{\mathrm{qdd}}\right)}{x_{l}-x_{\mathrm{qd}}}\right)}{x_{\mathrm{qdd}}}\right)}{{\left(x_{l}-x_{\mathrm{qd}}\right)}^2}\right)}{T_{\mathrm{qd}}}$
      | Automatically generated on 2025-10-31 19:34:58 .
  State_psi_gq_SG_D_2_a8fc7 : Inport
  State_psi_gq_SG_D_2_62489 : Inport  Port=2
  State_psi_kq_SG_D_2_c8166 : Inport  Port=3
  State_psi_gq_SG_D_2_800fa : Inport  Port=4
  State_psi_kq_SG_D_2_dce92 : Inport  Port=5
  State_psi_q_SG_D_2_7905a : Inport  Port=6
  State_psi_gq_SG_D_2_1a12c : Inport  Port=7
  State_psi_kq_SG_D_2_80d74 : Inport  Port=8
  State_psi_q_SG_D_2_b32ef : Inport  Port=9
  Add_06061 : Sum
  Add_14c97 : Sum
  Add_20850 : Sum
  Add_3ad81 : Sum
  Add_4f930 : Sum
  Add_6f9c6 : Sum
  Add_78547 : Sum
  Add_b8a05 : Sum
  Add_babc1 : Sum
  Add_dc432 : Sum
  Add_e76f3 : Sum
  Add_eeb16 : Sum
  Constant_-1_02cd3 : Constant  Value=-1
  Constant_-1_066dc : Constant  Value=-1
  Constant_-1_092ee : Constant  Value=-1
  Constant_-1_289da : Constant  Value=-1
  Constant_-1_3162f : Constant  Value=-1
  Constant_-1_7339d : Constant  Value=-1
  Constant_-1_a6a82 : Constant  Value=-1
  Constant_-1_b0314 : Constant  Value=-1
  Constant_-1_b9c05 : Constant  Value=-1
  Constant_-1_d8300 : Constant  Value=-1
  Constant_2.0_88f60 : Constant  Value=2.0
  Constant_T_qd_26db2 : Constant  Value=T_qd
  Constant_x_l_07494 : Constant  Value=x_l
  Constant_x_l_20257 : Constant  Value=x_l
  Constant_x_l_3c8be : Constant  Value=x_l
  Constant_x_l_43180 : Constant  Value=x_l
  Constant_x_l_4b5d1 : Constant  Value=x_l
  Constant_x_l_70261 : Constant  Value=x_l
  Constant_x_l_b454e : Constant  Value=x_l
  Constant_x_l_c0d58 : Constant  Value=x_l
  Constant_x_q_5f131 : Constant  Value=x_q
  Constant_x_qd_159ef : Constant  Value=x_qd
  Constant_x_qd_4324f : Constant  Value=x_qd
  Constant_x_qd_50591 : Constant  Value=x_qd
  Constant_x_qd_5c6fb : Constant  Value=x_qd
  Constant_x_qd_79022 : Constant  Value=x_qd
  Constant_x_qd_9a7eb : Constant  Value=x_qd
  Constant_x_qd_9ca23 : Constant  Value=x_qd
  Constant_x_qd_e190e : Constant  Value=x_qd
  Constant_x_qd_e1a4e : Constant  Value=x_qd
  Constant_x_qd_f7f60 : Constant  Value=x_qd
  Constant_x_qdd_2b66e : Constant  Value=x_qdd
  Constant_x_qdd_7a6f2 : Constant  Value=x_qdd
  Constant_x_qdd_97a87 : Constant  Value=x_qdd
  Constant_x_qdd_a134c : Constant  Value=x_qdd
  Constant_x_qdd_dd426 : Constant  Value=x_qdd
  Constant_x_qdd_de8f9 : Constant  Value=x_qdd
  Constant_x_qdd_fc116 : Constant  Value=x_qdd
  Divide_38f35 : Product  Inputs=*/
  Divide_5269d : Product  Inputs=*/
  Divide_7b1b6 : Product  Inputs=*/
  Divide_7f9e7 : Product  Inputs=*/
  Divide_88138 : Product  Inputs=*/
  Divide_98724 : Product  Inputs=*/
  Divide_a7233 : Product  Inputs=*/
  Divide_d56e2 : Product  Inputs=*/
  Power_4ea09 : Math  Operator=pow
  Product_0ccae : Product
  Product_240f3 : Product
  Product_24f45 : Product
  Product_3fa9d : Product
  Product_4c1f1 : Product
  Product_4da64 : Product
  Product_56d61 : Product
  Product_5c996 : Product
  Product_74ea4 : Product
  Product_7e381 : Product
  Product_802e2 : Product
  Product_a33c4 : Product
  Product_b5e40 : Product
  Product_b84a0 : Product
  Product_cde0c : Product
  Product_dc607 : Product
  Product_f4754 : Product
  Subtract_08f3c : Sum  Inputs=+-
  Subtract_1413c : Sum  Inputs=+-
  Subtract_20fd6 : Sum  Inputs=+-
  Subtract_420d3 : Sum  Inputs=+-
  Subtract_4d1dc : Sum  Inputs=+-
  Subtract_59b65 : Sum  Inputs=+-
  Subtract_8f8a0 : Sum  Inputs=+-
  Subtract_9fcbd : Sum  Inputs=+-
  Blockout_d_psi_gq_SG_D_2_b1325 : Outport
  wires:
  Constant_x_l_07494/1 -> Product_56d61/2
  Constant_x_l_c0d58/1 -> Product_a33c4/2
  Constant_x_qd_e1a4e/1 -> Subtract_8f8a0/1
  Constant_x_l_70261/1 -> Product_4c1f1/2
  Constant_x_qdd_2b66e/1 -> Subtract_420d3/2
  Constant_-1_d8300/1 -> Product_cde0c/1
  Constant_-1_7339d/1 -> Product_f4754/1
  State_psi_gq_SG_D_2_62489/1 -> Add_e76f3/1
  Constant_x_qdd_97a87/1 -> Subtract_8f8a0/2
  Constant_x_qd_4324f/1 -> Subtract_420d3/1
  Constant_x_l_4b5d1/1 -> Product_cde0c/2
  Constant_x_l_43180/1 -> Product_f4754/2
  Product_cde0c/1 -> Add_eeb16/1
  Product_f4754/1 -> Add_b8a05/1
  Constant_x_l_b454e/1 -> Product_5c996/2
  Constant_x_l_3c8be/1 -> Product_b84a0/2
  Constant_x_qd_159ef/1 -> Add_eeb16/2
  Constant_x_qdd_fc116/1 -> Add_b8a05/2
  Constant_-1_b9c05/1 -> Product_5c996/1
  Constant_x_qd_5c6fb/1 -> Add_6f9c6/2
  Constant_x_qdd_dd426/1 -> Add_20850/2
  State_psi_gq_SG_D_2_800fa/1 -> Product_802e2/1
  Add_eeb16/1 -> Divide_98724/2
  Add_b8a05/1 -> Product_802e2/2
  Constant_x_qd_e190e/1 -> Subtract_1413c/2
  Product_5c996/1 -> Add_dc432/1
  Constant_x_qd_f7f60/1 -> Add_dc432/2
  State_psi_kq_SG_D_2_dce92/1 -> Product_24f45/1
  Divide_a7233/1 -> Subtract_4d1dc/1
  Subtract_8f8a0/1 -> Product_24f45/2
  Product_802e2/1 -> Divide_a7233/1
  Add_dc432/1 -> Divide_a7233/2
  Add_78547/1 -> Product_3fa9d/2
  Product_24f45/1 -> Divide_98724/1
  Constant_-1_a6a82/1 -> Product_b84a0/1
  Divide_98724/1 -> Subtract_4d1dc/2
  Constant_-1_02cd3/1 -> Product_56d61/1
  Constant_-1_066dc/1 -> Product_a33c4/1
  Product_b84a0/1 -> Add_14c97/1
  Constant_x_qdd_a134c/1 -> Subtract_9fcbd/2
  Constant_x_qd_79022/1 -> Add_14c97/2
  Subtract_4d1dc/1 -> Add_78547/1
  Constant_-1_b0314/1 -> Product_4c1f1/1
  State_psi_q_SG_D_2_7905a/1 -> Add_78547/2
  Product_56d61/1 -> Add_6f9c6/1
  Product_a33c4/1 -> Add_20850/1
  Constant_-1_3162f/1 -> Product_dc607/1
  Product_3fa9d/1 -> Divide_38f35/1
  Constant_x_l_20257/1 -> Product_dc607/2
  Product_240f3/1 -> Add_babc1/2
  Constant_x_qd_9a7eb/1 -> Subtract_9fcbd/1
  Add_14c97/1 -> Product_3fa9d/1
  State_psi_gq_SG_D_2_1a12c/1 -> Product_4da64/1
  Add_6f9c6/1 -> Divide_88138/2
  Add_20850/1 -> Product_4da64/2
  Product_dc607/1 -> Add_4f930/1
  Constant_x_qd_50591/1 -> Add_4f930/2
  State_psi_kq_SG_D_2_80d74/1 -> Product_74ea4/1
  Subtract_9fcbd/1 -> Product_74ea4/2
  Divide_88138/1 -> Subtract_59b65/2
  State_psi_kq_SG_D_2_c8166/1 -> Add_e76f3/2
  Product_74ea4/1 -> Divide_88138/1
  Constant_x_qdd_7a6f2/1 -> Divide_38f35/2
  Product_4da64/1 -> Divide_5269d/1
  Add_4f930/1 -> Divide_5269d/2
  Constant_-1_092ee/1 -> Product_b5e40/1
  Subtract_420d3/1 -> Product_b5e40/2
  Add_e76f3/1 -> Subtract_20fd6/1
  Divide_38f35/1 -> Subtract_20fd6/2
  Product_4c1f1/1 -> Add_06061/1
  Constant_x_qd_9ca23/1 -> Add_06061/2
  Divide_5269d/1 -> Subtract_59b65/1
  Product_b5e40/1 -> Product_0ccae/1
  Subtract_20fd6/1 -> Product_0ccae/2
  Add_06061/1 -> Power_4ea09/1
  Constant_2.0_88f60/1 -> Power_4ea09/2
  Subtract_59b65/1 -> Add_3ad81/1
  State_psi_q_SG_D_2_b32ef/1 -> Add_3ad81/2
  Product_0ccae/1 -> Divide_7b1b6/1
  Power_4ea09/1 -> Divide_7b1b6/2
  Add_3ad81/1 -> Divide_7f9e7/1
  Constant_x_qdd_de8f9/1 -> Divide_7f9e7/2
  Constant_x_q_5f131/1 -> Subtract_1413c/1
  Divide_7b1b6/1 -> Subtract_08f3c/1
  Divide_7f9e7/1 -> Subtract_08f3c/2
  Divide_d56e2/1 -> Blockout_d_psi_gq_SG_D_2_b1325/1
  Constant_-1_289da/1 -> Product_7e381/1
  State_psi_gq_SG_D_2_a8fc7/1 -> Product_7e381/2
  Subtract_1413c/1 -> Product_240f3/1
  Subtract_08f3c/1 -> Product_240f3/2
  Product_7e381/1 -> Add_babc1/1
  Add_babc1/1 -> Divide_d56e2/1
  Constant_T_qd_26db2/1 -> Divide_d56e2/2

== system case9/Apparatus/SG_D_2/d_psi_kq_SG_D_2_block ==
  note: d_psi_kq_SG_D_2 in case9
      | $-\frac{\psi _{\mathrm{gq},\mathrm{SG},D,2}+\psi _{\mathrm{kq},\mathrm{SG},D,2}+\frac{\left(x_{l}-x_{\mathrm{qd}}\right)\,\left(\psi _{q,\mathrm{SG},D,2}+\frac{\psi _{\mathrm{gq},\mathrm{SG},D,2}\,\left(x_{l}-x_{\mathrm{qdd}}\right)}{x_{l}-x_{\mathrm{qd}}}+\frac{\psi _{\mathrm{kq},\mathrm{SG},D,2}\,\left(x_{\mathrm{qd}}-x_{\mathrm{qdd}}\right)}{x_{l}-x_{\mathrm{qd}}}\right)}{x_{\mathrm{qdd}}}}{T_{\mathrm{qdd}}}$
      | Automatically generated on 2025-10-31 19:34:59 .
  State_psi_gq_SG_D_2_04489 : Inport
  State_psi_kq_SG_D_2_1cb7b : Inport  Port=2
  State_psi_gq_SG_D_2_3c45c : Inport  Port=3
  State_psi_kq_SG_D_2_23860 : Inport  Port=4
  State_psi_q_SG_D_2_1b95e : Inport  Port=5
  Add_23d4e : Sum
  Add_5e4c1 : Sum
  Add_66db9 : Sum
  Add_b2c54 : Sum
  Add_e1730 : Sum
  Add_ed01d : Sum
  Constant_-1_07175 : Constant  Value=-1
  Constant_-1_2e0f4 : Constant  Value=-1
  Constant_-1_4a4d6 : Constant  Value=-1
  Constant_-1_719f3 : Constant  Value=-1
  Constant_-1_9745b : Constant  Value=-1
  Constant_T_qdd_a11f7 : Constant  Value=T_qdd
  Constant_x_l_34025 : Constant  Value=x_l
  Constant_x_l_40d47 : Constant  Value=x_l
  Constant_x_l_47673 : Constant  Value=x_l
  Constant_x_l_d4455 : Constant  Value=x_l
  Constant_x_qd_0f33d : Constant  Value=x_qd
  Constant_x_qd_18df6 : Constant  Value=x_qd
  Constant_x_qd_37516 : Constant  Value=x_qd
  Constant_x_qd_f4b47 : Constant  Value=x_qd
  Constant_x_qdd_9e8e9 : Constant  Value=x_qdd
  Constant_x_qdd_cd217 : Constant  Value=x_qdd
  Constant_x_qdd_de7ff : Constant  Value=x_qdd
  Divide_1f23b : Product  Inputs=*/
  Divide_251db : Product  Inputs=*/
  Divide_5aaa4 : Product  Inputs=*/
  Divide_81e0a : Product  Inputs=*/
  Product_12f1c : Product
  Product_2d13b : Product
  Product_2f349 : Product
  Product_7e043 : Product
  Product_b8d50 : Product
  Product_bc237 : Product
  Product_befa9 : Product
  Product_c9a6b : Product
  Subtract_5d84e : Sum  Inputs=+-
  Subtract_791f0 : Sum  Inputs=+-
  Subtract_94da8 : Sum  Inputs=+-
  Blockout_d_psi_kq_SG_D_2_396ab : Outport
  wires:
  State_psi_kq_SG_D_2_1cb7b/1 -> Subtract_791f0/2
  Constant_-1_07175/1 -> Product_befa9/1
  Constant_-1_2e0f4/1 -> Product_2d13b/1
  Constant_x_l_40d47/1 -> Product_2d13b/2
  Constant_x_qdd_cd217/1 -> Add_e1730/2
  Constant_x_l_34025/1 -> Product_befa9/2
  Constant_x_qd_18df6/1 -> Subtract_94da8/1
  Constant_T_qdd_a11f7/1 -> Divide_251db/2
  Constant_-1_4a4d6/1 -> Product_12f1c/1
  Product_2d13b/1 -> Add_e1730/1
  Constant_x_qdd_de7ff/1 -> Subtract_94da8/2
  Constant_x_l_d4455/1 -> Product_12f1c/2
  Divide_251db/1 -> Blockout_d_psi_kq_SG_D_2_396ab/1
  State_psi_gq_SG_D_2_3c45c/1 -> Product_c9a6b/1
  Add_e1730/1 -> Product_c9a6b/2
  Product_befa9/1 -> Add_b2c54/1
  Constant_x_qd_37516/1 -> Add_b2c54/2
  Product_7e043/1 -> Divide_81e0a/1
  State_psi_kq_SG_D_2_23860/1 -> Product_bc237/1
  Subtract_94da8/1 -> Product_bc237/2
  Product_12f1c/1 -> Add_23d4e/1
  Constant_x_qd_0f33d/1 -> Add_23d4e/2
  Product_bc237/1 -> Divide_5aaa4/1
  Product_c9a6b/1 -> Divide_1f23b/1
  Add_b2c54/1 -> Divide_1f23b/2
  Add_23d4e/1 -> Divide_5aaa4/2
  State_psi_q_SG_D_2_1b95e/1 -> Add_5e4c1/2
  Constant_-1_9745b/1 -> Product_b8d50/1
  Constant_x_l_47673/1 -> Product_b8d50/2
  Divide_1f23b/1 -> Subtract_5d84e/1
  Divide_5aaa4/1 -> Subtract_5d84e/2
  Product_b8d50/1 -> Add_66db9/1
  Constant_x_qd_f4b47/1 -> Add_66db9/2
  Subtract_5d84e/1 -> Add_5e4c1/1
  Constant_x_qdd_9e8e9/1 -> Divide_81e0a/2
  Constant_-1_719f3/1 -> Product_2f349/1
  State_psi_gq_SG_D_2_04489/1 -> Product_2f349/2
  Add_66db9/1 -> Product_7e043/1
  Add_5e4c1/1 -> Product_7e043/2
  Product_2f349/1 -> Subtract_791f0/1
  Subtract_791f0/1 -> Add_ed01d/1
  Divide_81e0a/1 -> Add_ed01d/2
  Add_ed01d/1 -> Divide_251db/1

== system case9/Apparatus/SG_D_2/d_psi_q_SG_D_2_block ==
  note: d_psi_q_SG_D_2 in case9
      | $2\,\pi \,f_{0}\,\left(v_{d,\mathrm{SG},D,2}\,\cos\left(\theta _{\mathrm{SG},D,2}\right)+v_{q,\mathrm{SG},D,2}\,\sin\left(\theta _{\mathrm{SG},D,2}\right)-\frac{R_{a}\,\left(\psi _{q,\mathrm{SG},D,2}+\frac{\psi _{\mathrm{gq},\mathrm{SG},D,2}\,\left(x_{l}-x_{\mathrm{qdd}}\right)}{x_{l}-x_{\mathrm{qd}}}+\frac{\psi _{\mathrm{kq},\mathrm{SG},D,2}\,\left(x_{\mathrm{qd}}-x_{\mathrm{qdd}}\right)}{x_{l}-x_{\mathrm{qd}}}\right)}{x_{\mathrm{qdd}}}-\frac{\psi _{d,\mathrm{SG},D,2}\,w_{\mathrm{SG},D,2}}{2\,f_{0}\,\pi }\right)$
      | Automatically generated on 2025-10-31 19:34:55 .
  State_psi_gq_SG_D_2_67ca3 : Inport
  State_psi_kq_SG_D_2_eff29 : Inport  Port=2
  State_psi_q_SG_D_2_2e7f8 : Inport  Port=3
  Input_v_d_SG_D_2_67ef1 : Inport  Port=4
  State_theta_SG_D_2_cc426 : Inport  Port=5
  Input_v_q_SG_D_2_8572d : Inport  Port=6
  State_theta_SG_D_2_a97e0 : Inport  Port=7
  State_psi_d_SG_D_2_78148 : Inport  Port=8
  State_w_SG_D_2_cdc87 : Inport  Port=9
  Add_20e73 : Sum
  Add_58493 : Sum
  Add_5f1f5 : Sum
  Add_a4deb : Sum
  Add_aea06 : Sum
  Constant_-1_170e5 : Constant  Value=-1
  Constant_-1_632c8 : Constant  Value=-1
  Constant_-1_f9f92 : Constant  Value=-1
  Constant_-2.0_db6e8 : Constant  Value=-2.0
  Constant_2.0_2f7be : Constant  Value=2.0
  Constant_R_a_aab2d : Constant  Value=R_a
  Constant_f0_26ab5 : Constant  Value=f0
  Constant_f0_faaa6 : Constant  Value=f0
  Constant_pi_8c890 : Constant  Value=pi
  Constant_pi_bd9ab : Constant  Value=pi
  Constant_x_l_39787 : Constant  Value=x_l
  Constant_x_l_61f4c : Constant  Value=x_l
  Constant_x_l_d6606 : Constant  Value=x_l
  Constant_x_qd_3274b : Constant  Value=x_qd
  Constant_x_qd_71907 : Constant  Value=x_qd
  Constant_x_qd_8f591 : Constant  Value=x_qd
  Constant_x_qdd_19646 : Constant  Value=x_qdd
  Constant_x_qdd_87955 : Constant  Value=x_qdd
  Constant_x_qdd_dc605 : Constant  Value=x_qdd
  Divide_69fd9 : Product  Inputs=*/
  Divide_992a0 : Product  Inputs=*/
  Divide_d6c00 : Product  Inputs=*/
  Divide_f38f8 : Product  Inputs=*/
  MathFunc_cos_ca799 : Trigonometry  Operator=cos
  MathFunc_sin_79341 : Trigonometry
  Product_0b3ea : Product
  Product_0b897 : Product
  Product_366a0 : Product
  Product_3fb4c : Product
  Product_42562 : Product
  Product_431f3 : Product
  Product_4c5c1 : Product
  Product_6ab33 : Product
  Product_7746f : Product
  Product_82ba4 : Product
  Product_bedf7 : Product
  Product_d8867 : Product
  Product_e5bde : Product
  Product_e837f : Product
  Subtract_2be2a : Sum  Inputs=+-
  Subtract_391a7 : Sum  Inputs=+-
  Subtract_7c0da : Sum  Inputs=+-
  Subtract_d1cbc : Sum  Inputs=+-
  Blockout_d_psi_q_SG_D_2_f15c9 : Outport
  wires:
  Constant_x_qdd_dc605/1 -> Subtract_2be2a/2
  Constant_x_l_d6606/1 -> Product_e5bde/2
  Constant_-1_632c8/1 -> Product_431f3/1
  Constant_x_l_61f4c/1 -> Product_431f3/2
  Product_431f3/1 -> Add_20e73/1
  Constant_pi_8c890/1 -> Product_0b897/2
  State_psi_gq_SG_D_2_67ca3/1 -> Product_3fb4c/1
  Constant_x_l_39787/1 -> Product_366a0/2
  State_w_SG_D_2_cdc87/1 -> Product_e837f/2
  Constant_x_qd_71907/1 -> Add_aea06/2
  Constant_x_qdd_87955/1 -> Add_20e73/2
  Constant_2.0_2f7be/1 -> Product_0b897/1
  Constant_-1_170e5/1 -> Product_366a0/1
  Constant_x_qd_8f591/1 -> Subtract_2be2a/1
  Constant_-1_f9f92/1 -> Product_e5bde/1
  State_psi_q_SG_D_2_2e7f8/1 -> Add_a4deb/2
  Add_20e73/1 -> Product_3fb4c/2
  Product_0b897/1 -> Product_bedf7/1
  Product_366a0/1 -> Add_5f1f5/1
  Constant_pi_bd9ab/1 -> Product_42562/2
  Constant_f0_faaa6/1 -> Product_bedf7/2
  Constant_x_qd_3274b/1 -> Add_5f1f5/2
  State_psi_kq_SG_D_2_eff29/1 -> Product_7746f/1
  Subtract_2be2a/1 -> Product_7746f/2
  Product_e5bde/1 -> Add_aea06/1
  Input_v_q_SG_D_2_8572d/1 -> Product_0b3ea/1
  Product_3fb4c/1 -> Divide_d6c00/1
  Product_bedf7/1 -> Divide_992a0/2
  Add_5f1f5/1 -> Divide_d6c00/2
  Product_7746f/1 -> Divide_69fd9/1
  Add_aea06/1 -> Divide_69fd9/2
  Divide_d6c00/1 -> Subtract_7c0da/1
  State_theta_SG_D_2_cc426/1 -> MathFunc_cos_ca799/1
  Divide_69fd9/1 -> Subtract_7c0da/2
  Subtract_7c0da/1 -> Add_a4deb/1
  MathFunc_cos_ca799/1 -> Product_d8867/2
  Constant_R_a_aab2d/1 -> Product_82ba4/1
  Add_a4deb/1 -> Product_82ba4/2
  State_theta_SG_D_2_a97e0/1 -> MathFunc_sin_79341/1
  Product_82ba4/1 -> Divide_f38f8/1
  Product_42562/1 -> Product_6ab33/1
  Product_0b3ea/1 -> Subtract_d1cbc/2
  Constant_x_qdd_19646/1 -> Divide_f38f8/2
  Input_v_d_SG_D_2_67ef1/1 -> Product_d8867/1
  Add_58493/1 -> Product_4c5c1/2
  Divide_f38f8/1 -> Subtract_391a7/1
  Product_d8867/1 -> Subtract_391a7/2
  MathFunc_sin_79341/1 -> Product_0b3ea/2
  Product_4c5c1/1 -> Blockout_d_psi_q_SG_D_2_f15c9/1
  State_psi_d_SG_D_2_78148/1 -> Product_e837f/1
  Constant_-2.0_db6e8/1 -> Product_42562/1
  Product_6ab33/1 -> Product_4c5c1/1
  Subtract_391a7/1 -> Subtract_d1cbc/1
  Product_e837f/1 -> Divide_992a0/1
  Constant_f0_26ab5/1 -> Product_6ab33/2
  Subtract_d1cbc/1 -> Add_58493/1
  Divide_992a0/1 -> Add_58493/2

== system case9/Apparatus/SG_D_2/d_theta_SG_D_2_block ==
  note: d_theta_SG_D_2 in case9
      | $w_{\mathrm{SG},D,2}-2\,\pi \,f_{0}$
      | Automatically generated on 2025-10-31 19:35:00 .
  State_w_SG_D_2_c3833 : Inport
  Add_96360 : Sum
  Constant_-2.0_f8c9e : Constant  Value=-2.0
  Constant_f0_6ca16 : Constant  Value=f0
  Constant_pi_61c1d : Constant  Value=pi
  Product_3db73 : Product
  Product_abea2 : Product
  Blockout_d_theta_SG_D_2_999e7 : Outport
  wires:
  Constant_-2.0_f8c9e/1 -> Product_abea2/1
  Constant_pi_61c1d/1 -> Product_abea2/2
  Add_96360/1 -> Blockout_d_theta_SG_D_2_999e7/1
  Product_abea2/1 -> Product_3db73/1
  Constant_f0_6ca16/1 -> Product_3db73/2
  Product_3db73/1 -> Add_96360/1
  State_w_SG_D_2_c3833/1 -> Add_96360/2
